simulink model "Control_sim_FixedV"  (R2023b)
settings: Solver=ode3  StartTime=0.0  StopTime=50  FixedStep=0.05  RelTol=1e-3  EnableMultiTasking=on
values from neighbouring files (symbols this model uses):
  k_alpha = 11    [parameters.m]
  kdalpha = 0    [parameters.m]
  ki_alpha = 22    [Simulation_code.m]    (also in parameters.m = 0)
  theta0 = theta    (= 4.71238898038)    [Simulation_code.m]    (also in parameters.m = -1.57079632679)
  tol = 0.02    [Simulation_code.m]    (also in parameters.m)
  v = Vmax    (= 0.8)    [Simulation_code.m]    (also in parameters.m)
  Wmax = 3    [Simulation_code.m]    (also in parameters.m)
  xg = 5    [Simulation_code.m]    (also in parameters.m)
  yg = 5    [Simulation_code.m]    (also in parameters.m)
libraries: slpidlib x1
settings Model: Creator=Shaam  LastModifiedBy=Hadi
settings SolverCC: AlgebraicLoopSolver=TrustRegion
settings DataIOCC: LimitDataPoints=on  SaveFormat=Array  ReturnWorkspaceOutputs=off
settings OptimizationCC: LifeSpan=inf
settings DebuggingCC: UnderspecifiedInitializationDetection=Classic  MergeDetectMultiDrivingBlocksExec=none  SolverPrmCheckMsg=warning  UnconnectedInputMsg=warning  UnconnectedOutputMsg=warning  UnconnectedLineMsg=warning  StateNameClashWarn=warning  SFUnexpectedBacktrackingDiag=warning  SFNoUnconditionalDefaultTransitionDiag=warning  SFExecutionAtInitializationDiag=none  ArithmeticOperatorsInVariantConditions=warning
settings HardwareCC: ProdBitPerPointer=32  ProdBitPerSizeT=32  ProdBitPerPtrDiffT=32  ProdLargestAtomicFloat=None  ProdIntDivRoundTo=Undefined  ProdEndianess=Unspecified  ProdWordSize=32  ProdHWDeviceType=32-bit Generic
settings ModelReferenceCC: PropagateSignalLabelsOutOfModel=off
settings SFSimCC: SimUseLocalCustomCode=off  CustomCodeUndefinedFunction=UseInterfaceOnly
settings RTWCC: RTWUseLocalCustomCode=off
settings CodeAppCC: StateflowObjectComments=on
settings GRTTargetCC: TargetLangStandard=C89/C90 (ANSI)
settings ConfigComp: CovMetricSettings=dw  CovSaveCumulativeToWorkspaceVar=on  CovSaveSingleToWorkspaceVar=on  CovExternalEMLEnable=off

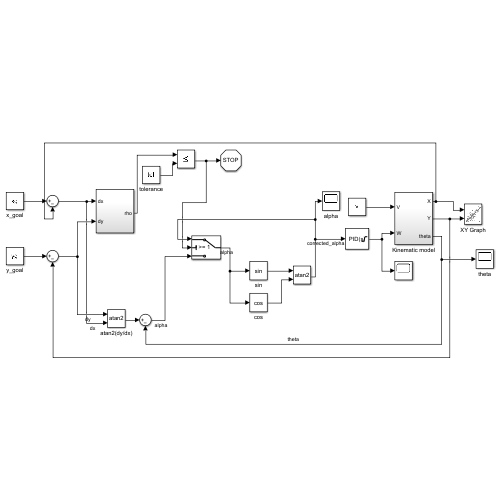
[thumbnail: Simulink's stored preview of the top-level diagram]
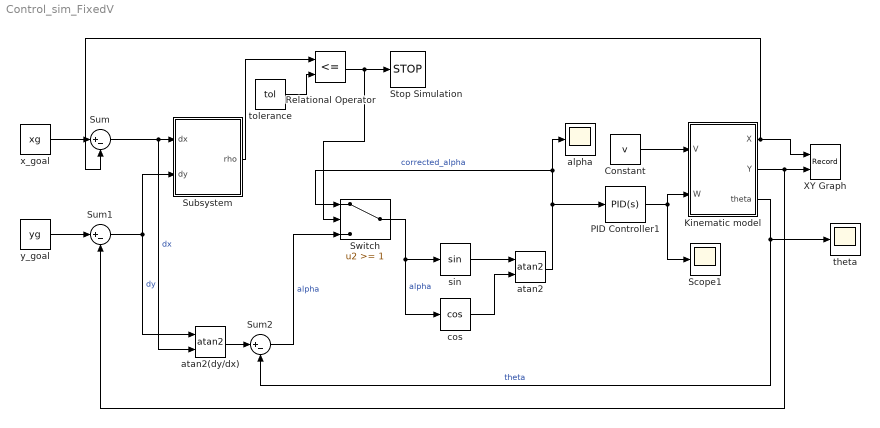
== system Control_sim_FixedV ==
  Constant : Constant  Value=v
  Kinematic model : Subsystem
  PID Controller1 : slpidlib/PID Controller  Controller=PID  Form=Parallel  TimeDomain=Continuous-time  UseExternalTs=off  SampleTime=1  IntegratorMethod=Forward Euler  FilterMethod=Forward Euler  ControllerParametersSource=internal  P=k_alpha  I=ki_alpha  UseKiTs=off  D=kdalpha  N=1  UseFilter=on  TunerSelectOption=Transfer Function Based (PID Tuner App)  InitialConditionSource=internal  InitialConditionForIntegrator=0  InitialConditionForFilter=0  DifferentiatorICPrevScaledInput=0  ExternalReset=none  TrackingMode=off  Kt=1  LimitOutput=on  SatLimitsSource=internal  UpperSaturationLimit=Wmax  LowerSaturationLimit=-Wmax  LinearizeAsGain=on  AntiWindupMode=none  Kb=1  LimitIntegrator=off  UpperIntegratorSaturationLimit=inf  LowerIntegratorSaturationLimit=-inf  POutMin=[]  POutMax=[]  IOutMin=[]  IOutMax=[]  DOutMin=[]  DOutMax=[]  NOutMin=[]  NOutMax=[]  SumOutMin=[]  SumOutMax=[]  SaturationOutMin=[]  SaturationOutMax=[]  PParamMin=[]  PParamMax=[]  IParamMin=[]  IParamMax=[]  DParamMin=[]  DParamMax=[]  NParamMin=[]  NParamMax=[]  KbParamMin=[]  KbParamMax=[]  KtParamMin=[]  KtParamMax=[]  KbOutMin=[]  KbOutMax=[]  KtOutMin=[]  KtOutMax=[]  IntegratorOutMin=[]  IntegratorOutMax=[]  FilterOutMin=[]  FilterOutMax=[]  SumI1OutMin=[]  SumI1OutMax=[]  SumI2OutMin=[]  SumI2OutMax=[]  SumI3OutMin=[]  SumI3OutMax=[]  SumI4OutMin=[]  SumI4OutMax=[]  SumDOutMin=[]  SumDOutMax=[]  DifferentiatorOutMin=[]  DifferentiatorOutMax=[]  FilterDiffOutCoefMin=[]  FilterDiffOutCoefMax=[]  ReciprocalOutMin=[]  ReciprocalOutMax=[]  SumDenOutMin=[]  SumDenOutMax=[]  SumNumOutMin=[]  SumNumOutMax=[]  DivideOutMin=[]  DivideOutMax=[]  UdiffTsProdOutMin=[]  UdiffTsProdOutMax=[]  NTsProdOutMin=[]  NTsProdOutMax=[]  UintegralTsProdOutMin=[]  UintegralTsProdOutMax=[]  UngainTsProdOutMin=[]  UngainTsProdOutMax=[]  ClampingZeroOutDataTypeStr=Inherit: Inherit via back propagation  ClampingZeroOutMin=[]  ClampingZeroOutMax=[]  FilterDenConstantOutDataTypeStr=Inherit: Inherit via back propagation  FilterDenConstantOutMin=[]  FilterDenConstantOutMax=[]  PCopyOutDataTypeStr=Inherit: Inherit via back propagation  PCopyOutMin=[]  PCopyOutMax=[]  NCopyOutDataTypeStr=Inherit: Inherit via back propagation  NCopyOutMin=[]  NCopyOutMax=[]  IntegratorContinuousStateAttributes=''  IntegratorStateMustResolveToSignalObject=off  IntegratorRTWStateStorageClass=Auto  FilterContinuousStateAttributes=''  FilterStateMustResolveToSignalObject=off  FilterRTWStateStorageClass=Auto  ParallelPVariant=InternalParameters  IdealPVariant=Disabled  IVariant=InternalParameters  DVariant=InternalParameters  IntegratorVariant=Continuous  SatVariant=Enabled  AWVariant=Passthrough  PCopyVariant=Disabled  TRVariant=Disabled  FdbkBlocksVariant=Forward  IdealPFdbkVariant=Disabled  SatFdbkVariant=Disabled  DerivativeFilterVariant=ContFilter  NVariant=InternalParameters  NCopyVariant=Disabled  FilterICVariant=InternalICsFilter  IntegratorICVariant=InternalICs  ExternalResetVariant=Disabled  TRSumVariant=Passthrough  SumFdbkVariant=Disabled  SumVariant=Sum_PID  TsampFilterVariant=InternalTs  TsampNgainVariant=Passthrough  TsampIntegralVariant=Disabled_SignalSpec  ExternalSaturationOutDataTypeStr=Inherit: Same as second input
  Relational Operator : RelationalOperator  Operator=<=  OutDataTypeStr=boolean  InputSameDT=off
  Scope1 : Scope
  Stop Simulation : Stop
  Subsystem : Subsystem
  Sum : Sum  Inputs=|+-
  Sum1 : Sum  Inputs=|+-
  Sum2 : Sum  Inputs=|+-
  Switch : Switch  Threshold=1  SaturateOnIntegerOverflow=off  InputSameDT=off
  XY Graph : Record  FileSettingsInternal="{\"entries\":[{\"content\":{\"excelSettings\":{\"content\":{},\"type\":\"Streamout.ExcelSettings\"}},\"type\":\"Streamout.FileSettingStorage\",\"uuid\":\"\"}],\"packageUris\":[\"http:\\/\\/schema.mathworks.com\\/mf0\\/streamout_blocks\\/R2020a\"],\"version\":\"1.0\"}"  Layout=[1 1]  SignalsInternal="{\"entries\":[{\"content\":{\"signals\":[{\"content\":{\"blockPath\":[],\"dimensions\":[1],\"domain\":\"\",\"lineColor\":\"#a2142f\",\"plots\":[1],\"port\":1,\"signalID\":8,\"signalName\":\"Kinematic model:1\"},\"type\":\"RecordBlkView.Signal\",\"uuid\":\"\"},{\"content\":{\"blockPath\":[],\"dimensions\":[1],\"domain\":\"\",\"lineColor\":\"#139fff\",\"plots\":[1],\"port\":2,\"signalID\":11,\"signalName\":\"Kinematic model:2\"},\"type\":\"RecordBlkView.Signal\",\"uuid\":\"\"}]},\"type\":\"RecordBlkView.InputSignals\",\"uuid\":\"\"}],\"packageUris\":[\"http:\\/\\/schema.mathworks.com\\/mf0\\/streamout_blocks\\/R2020a\"],\"version\":\"1.0\"}"  VisualizationBindings="{\"xyplotplugin\":{\"info\":[{\"series\":[{\"bindingParametersList\":[{\"parameter\":\"X-Axis\",\"signalID\":8,\"signalName\":\"Kinematic model:1\"},{\"parameter\":\"Y-Axis\",\"signalID\":11,\"signalName\":\"Kinematic model:2\"}],\"seriesID\":7776}],\"subplotID\":1}]}}"  CompatibilityTag=XY  st=-1
  alpha : Scope
  atan2 : Trigonometry  Operator=atan2
  atan2(dy/dx) : Trigonometry  Operator=atan2
  cos : Trigonometry  Operator=cos
  sin : Trigonometry
  theta : Scope
  tolerance : Constant  Value=tol
  x_goal : Constant  Value=xg
  y_goal : Constant  Value=yg
  wires:
  Kinematic model/1(X) -> Sum/2, XY Graph/1
  Kinematic model/2(Y) -> XY Graph/2, Sum1/2
  Kinematic model/3(theta) -> theta/1, Sum2/2  "theta"
  x_goal/1 -> Sum/1
  y_goal/1 -> Sum1/1
  Sum1/1 -> Subsystem/2(dy), atan2(dy/dx)/1  "dy"
  Sum/1 -> atan2(dy/dx)/2, Subsystem/1(dx)  "dx"
  Subsystem/1(rho) -> Relational Operator/1
  Sum2/1 -> Switch/3  "alpha"
  PID Controller1/1 -> Kinematic model/2(W), Scope1/1
  Constant/1 -> Kinematic model/1(V)
  tolerance/1 -> Relational Operator/2
  Relational Operator/1 -> Switch/2, Stop Simulation/1
  atan2(dy/dx)/1 -> Sum2/1
  sin/1 -> atan2/1
  cos/1 -> atan2/2
  atan2/1 -> alpha/1, Switch/1, PID Controller1/1  "corrected_alpha"
  Switch/1 -> cos/1, sin/1  "alpha"

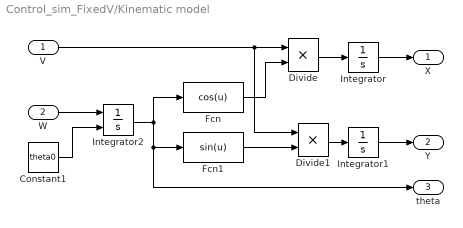
== system Control_sim_FixedV/Kinematic model ==
  V : Inport
  W : Inport  Port=2
  Constant1 : Constant  Value=theta0
  Divide : Product  Inputs=**
  Divide1 : Product  Inputs=**
  Fcn : Fcn  Expr=cos(u)
  Fcn1 : Fcn  Expr=sin(u)
  Integrator : Integrator
  Integrator1 : Integrator
  Integrator2 : Integrator  InitialConditionSource=external
  X : Outport
  Y : Outport  Port=2
  theta : Outport  Port=3
  wires:
  V/1 -> Divide1/1, Divide/1
  W/1 -> Integrator2/1
  Integrator2/1 -> theta/1, Fcn1/1, Fcn/1
  Divide1/1 -> Integrator1/1
  Fcn/1 -> Divide/2
  Divide/1 -> Integrator/1
  Integrator1/1 -> Y/1
  Integrator/1 -> X/1
  Fcn1/1 -> Divide1/2
  Constant1/1 -> Integrator2/2

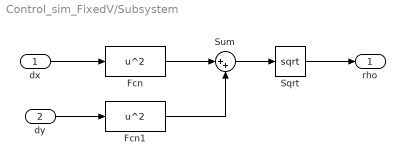
== system Control_sim_FixedV/Subsystem ==
  dx : Inport
  dy : Inport  Port=2
  Fcn : Fcn  Expr=u^2
  Fcn1 : Fcn  Expr=u^2
  Sqrt : Sqrt
  Sum : Sum  Inputs=|++
  rho : Outport
  wires:
  dy/1 -> Fcn1/1
  Sqrt/1 -> rho/1
  Fcn1/1 -> Sum/2
  Fcn/1 -> Sum/1
  Sum/1 -> Sqrt/1
  dx/1 -> Fcn/1
